simulink model "if_else"  (R2014a)
settings: Solver=ode45  StartTime=0.0  StopTime=10.0  RelTol=1e-3
settings Model: Creator=RANGA  LastModifiedBy=RANGA

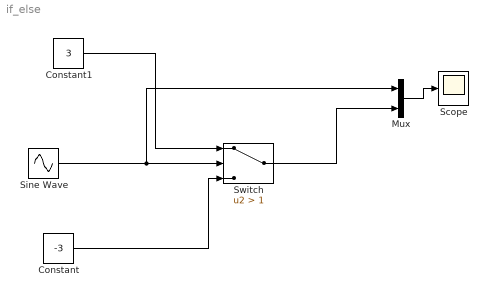
== system if_else ==
  Constant : Constant  Value=-3
  Constant1 : Constant  Value=3
  Mux : Mux  Inputs=2
  Scope : Scope
  Sine Wave : Sin  Amplitude=2  SampleTime=0
  Switch : Switch  Criteria=u2 > Threshold  Threshold=1
  wires:
  Sine Wave/1 -> Mux/1, Switch/2
  Constant1/1 -> Switch/1
  Constant/1 -> Switch/3
  Mux/1 -> Scope/1
  Switch/1 -> Mux/2
